simulink model "Motor_Pos"  (R2020a)
settings: Solver=ode45  StartTime=0.0  StopTime=0.2  RelTol=1e-3
model workspace (MAT data in the model file):
  K = 0.0274
undefined symbols (not defined in the file or in its folder): Kd, Ki, Kp
settings Model: DataDictionary=motor.sldd  Creator=sansh  LastModifiedBy=Admin
settings DataIOCC: ReturnWorkspaceOutputs=off
settings DebuggingCC: ArithmeticOperatorsInVariantConditions=warning
settings SFSimCC: SimUseLocalCustomCode=off  CustomCodeUndefinedFunction=UseInterfaceOnly
settings RTWCC: RTWUseLocalCustomCode=off
settings CodeAppCC: StateflowObjectComments=on

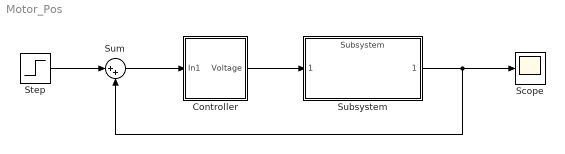
== system Motor_Pos ==
  Controller : Subsystem
  Scope : Scope
  Step : Step  SampleTime=0
  Subsystem : ModelReference  ModelNameDialog=Subsystem  ModelReferenceVersion=1.10
  Sum : Sum  Inputs=|++
  wires:
  Sum/1 -> Controller/1(In1)
  Step/1 -> Sum/1
  Subsystem/1 -> Sum/2, Scope/1
  Controller/1(Voltage) -> Subsystem/1

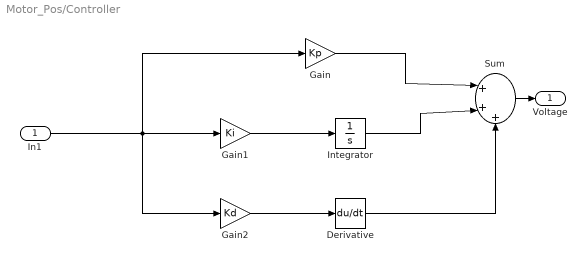
== system Motor_Pos/Controller ==
  In1 : Inport
  Derivative : Derivative
  Gain : Gain  Gain=Kp
  Gain1 : Gain  Gain=Ki
  Gain2 : Gain  Gain=Kd
  Integrator : Integrator
  Sum : Sum  Inputs=|+++
  Voltage : Outport
  wires:
  Gain/1 -> Sum/1
  In1/1 -> Gain2/1, Gain1/1, Gain/1
  Sum/1 -> Voltage/1
  Gain1/1 -> Integrator/1
  Gain2/1 -> Derivative/1
  Integrator/1 -> Sum/2
  Derivative/1 -> Sum/3
